simulink model "cranecontroller"  (R2025b)
settings: Solver=VariableStepAuto  StartTime=0.0  StopTime=3.5  RelTol=1e-3
libraries: slpidlib x1
settings Model: Creator=maliha  LastModifiedBy=maliha

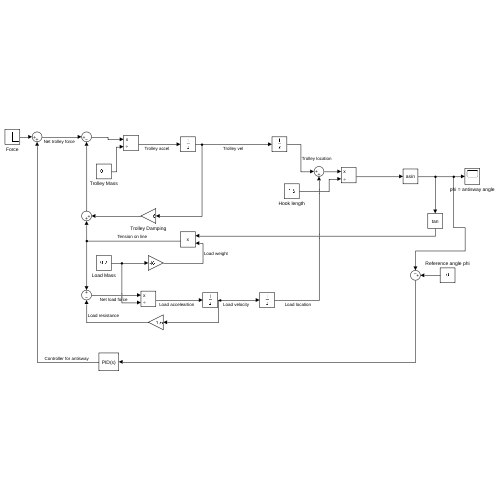
[thumbnail: Simulink's stored preview of the top-level diagram]
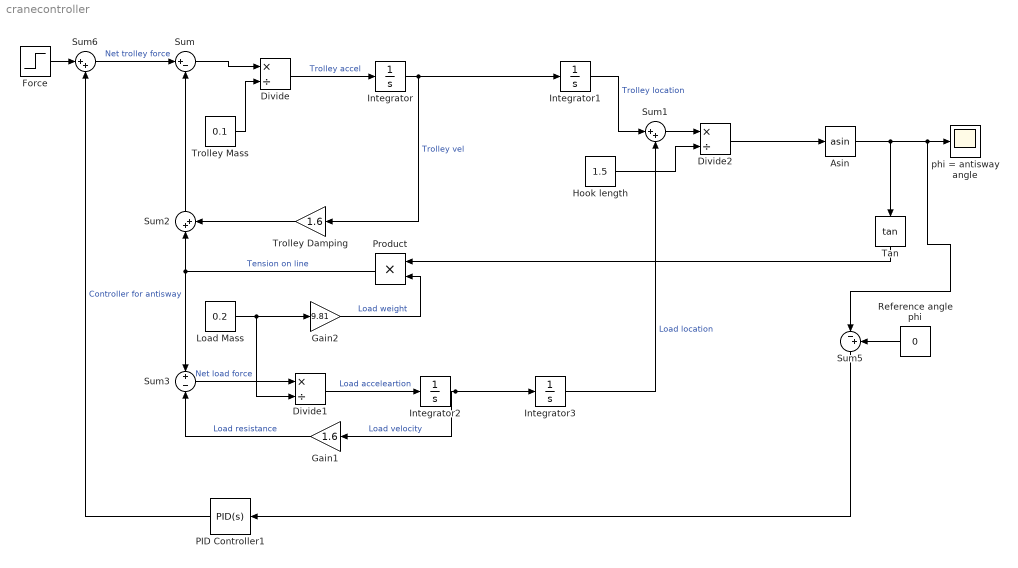
== system cranecontroller ==
  Asin : Trigonometry  Operator=asin
  Divide : Product  Inputs=*/
  Divide1 : Product  Inputs=*/
  Divide2 : Product  Inputs=*/
  Force : Step  Before=1  After=0  SampleTime=0
  Gain1 : Gain  Gain=1.6
  Gain2 : Gain  Gain=9.81
  Hook length : Constant  Value=1.5
  Integrator{,1..3} (4 alike) : Integrator
  Load Mass : Constant  Value=0.2
  PID Controller1 : slpidlib/PID Controller  Controller=PID  Form=Parallel  TimeDomain=Continuous-time  UseExternalTs=off  SampleTime=-1  IntegratorMethod=Forward Euler  FilterMethod=Forward Euler  ControllerParametersSource=internal  P=20  I=0  UseKiTs=off  D=0  UseExternalDerivativeSource=off  N=100  UseFilter=on  TunerSelectOption=Transfer Function Based (PID Tuner App)  InitialConditionSource=internal  InitialConditionForIntegrator=0  InitialConditionForFilter=0  DifferentiatorICPrevScaledInput=0  ExternalReset=none  TrackingMode=off  Kt=1  LimitOutput=off  SatLimitsSource=internal  UpperSaturationLimit=inf  LowerSaturationLimit=-inf  LinearizeAsGain=on  AntiWindupMode=none  Kb=1  LimitIntegrator=off  UpperIntegratorSaturationLimit=inf  LowerIntegratorSaturationLimit=-inf  POutMin=[]  POutMax=[]  IOutMin=[]  IOutMax=[]  DOutMin=[]  DOutMax=[]  NOutMin=[]  NOutMax=[]  SumOutMin=[]  SumOutMax=[]  SaturationOutMin=[]  SaturationOutMax=[]  PParamMin=[]  PParamMax=[]  IParamMin=[]  IParamMax=[]  DParamMin=[]  DParamMax=[]  NParamMin=[]  NParamMax=[]  KbParamMin=[]  KbParamMax=[]  KtParamMin=[]  KtParamMax=[]  KbOutMin=[]  KbOutMax=[]  KtOutMin=[]  KtOutMax=[]  IntegratorOutMin=[]  IntegratorOutMax=[]  FilterOutMin=[]  FilterOutMax=[]  SumI1OutMin=[]  SumI1OutMax=[]  SumI2OutMin=[]  SumI2OutMax=[]  SumI3OutMin=[]  SumI3OutMax=[]  SumI4OutMin=[]  SumI4OutMax=[]  SumDOutMin=[]  SumDOutMax=[]  DifferentiatorOutMin=[]  DifferentiatorOutMax=[]  FilterDiffOutCoefMin=[]  FilterDiffOutCoefMax=[]  ReciprocalOutMin=[]  ReciprocalOutMax=[]  SumDenOutMin=[]  SumDenOutMax=[]  SumNumOutMin=[]  SumNumOutMax=[]  DivideOutMin=[]  DivideOutMax=[]  UdiffTsProdOutMin=[]  UdiffTsProdOutMax=[]  NTsProdOutMin=[]  NTsProdOutMax=[]  UintegralTsProdOutMin=[]  UintegralTsProdOutMax=[]  UngainTsProdOutMin=[]  UngainTsProdOutMax=[]  ClampingZeroOutDataTypeStr=Inherit: Inherit via back propagation  ClampingZeroOutMin=[]  ClampingZeroOutMax=[]  FilterDenConstantOutDataTypeStr=Inherit: Inherit via back propagation  FilterDenConstantOutMin=[]  FilterDenConstantOutMax=[]  PCopyOutDataTypeStr=Inherit: Inherit via back propagation  PCopyOutMin=[]  PCopyOutMax=[]  NCopyOutDataTypeStr=Inherit: Inherit via back propagation  NCopyOutMin=[]  NCopyOutMax=[]  IntegratorContinuousStateAttributes=''  IntegratorStateMustResolveToSignalObject=off  IntegratorRTWStateStorageClass=Auto  FilterContinuousStateAttributes=''  FilterStateMustResolveToSignalObject=off  FilterRTWStateStorageClass=Auto  ParallelPVariant=InternalParameters  IdealPVariant=Disabled  IVariant=InternalParameters  DVariant=InternalParameters  IntegratorVariant=Continuous  SatVariant=Disabled  AWVariant=Passthrough  PCopyVariant=Disabled  TRVariant=Disabled  FdbkBlocksVariant=Forward  IdealPFdbkVariant=Disabled  SatFdbkVariant=Disabled  DerivativeFilterVariant=ContFilter  NVariant=InternalParameters  NCopyVariant=Disabled  FilterICVariant=InternalICsFilter  IntegratorICVariant=InternalICs  ExternalResetVariant=Disabled  TRSumVariant=Passthrough  SumFdbkVariant=Disabled  SumVariant=Sum_PID  TsampFilterVariant=InternalTs  TsampNgainVariant=Passthrough  TsampIntegralVariant=Disabled_SignalSpec  ExternalSaturationOutDataTypeStr=Inherit: Same as second input  DerivativeSourceVariant=ErrorSignal  PreIntVariant=InternalPreInt
  Product : Product
  Reference angle phi : Constant  Value=0
  Sum : Sum  Inputs=|+-
  Sum1 : Sum  Inputs=|++
  Sum2 : Sum  Inputs=|++
  Sum3 : Sum  Inputs=+|-
  Sum5 : Sum  Inputs=|-+
  Sum6 : Sum  Inputs=|++
  Tan : Trigonometry  Operator=tan
  Trolley Damping : Gain  Gain=1.6
  Trolley Mass : Constant  Value=0.1
  phi = antisway angle : Scope
      settings: ActiveDisplayYMinimum=-0.0082136444862271323  ActiveDisplayYMaximum=0.058137069381661417
  wires:
  Sum/1 -> Divide/1
  Divide/1 -> Integrator/1  "Trolley accel"
  Integrator/1 -> Trolley Damping/1, Integrator1/1  "Trolley vel"
  Integrator1/1 -> Sum1/1  "Trolley location"
  Trolley Mass/1 -> Divide/2
  Sum2/1 -> Sum/2
  Gain1/1 -> Sum3/2  "Load resistance"
  Sum3/1 -> Divide1/1  "Net load force"
  Divide1/1 -> Integrator2/1  "Load acceleartion"
  Integrator2/1 -> Gain1/1, Integrator3/1  "Load velocity"
  Integrator3/1 -> Sum1/2  "Load location"
  Load Mass/1 -> Gain2/1, Divide1/2
  Gain2/1 -> Product/2  "Load weight"
  Product/1 -> Sum3/1, Sum2/1  "Tension on line"
  Sum1/1 -> Divide2/1
  Hook length/1 -> Divide2/2
  Divide2/1 -> Asin/1
  Asin/1 -> Sum5/1, phi = antisway angle/1, Tan/1
  Tan/1 -> Product/1
  Trolley Damping/1 -> Sum2/2
  Force/1 -> Sum6/1
  Sum5/1 -> PID Controller1/1
  Reference angle phi/1 -> Sum5/2
  PID Controller1/1 -> Sum6/2  "Controller for antisway"
  Sum6/1 -> Sum/1  "Net trolley force"
